simulink model "FM"  (R2018b)
settings: Solver=VariableStepAuto  StartTime=0.0  StopTime=10.0  MaxStep=0.001  RelTol=1e-3
libraries: commanapbnd3 x1
settings Model: Creator=sin  LastModifiedBy=sin

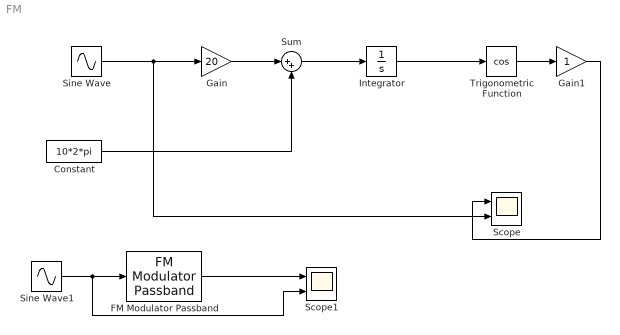
== system FM ==
  Constant : Constant  Value=10*2*pi
  FM Modulator Passband : commanapbnd3/FM Modulator Passband  Fc=10  Ph=0  Kc=5
      settings: SourceProductName=Communications System Toolbox  SourceProductBaseCode=CM
  Gain : Gain  Gain=20
  Gain1 : Gain
  Integrator : Integrator
  Scope : Scope  NumInputPorts=2
  Scope1 : Scope  NumInputPorts=2
  Sine Wave : Sin  Frequency=1*2*pi  SampleTime=0
  Sine Wave1 : Sin  Frequency=1*2*pi  SampleTime=0.001
  Sum : Sum  Inputs=|++
  Trigonometric Function : Trigonometry  Operator=cos
  wires:
  Gain/1 -> Sum/1
  Sine Wave/1 -> Scope/2, Gain/1
  Constant/1 -> Sum/2
  Sum/1 -> Integrator/1
  Integrator/1 -> Trigonometric Function/1
  Trigonometric Function/1 -> Gain1/1
  Gain1/1 -> Scope/1
  Sine Wave1/1 -> Scope1/2, FM Modulator Passband/1
  FM Modulator Passband/1 -> Scope1/1
